simulink model "community_charts"  (R2018a)
settings: Solver=VariableStepAuto  StartTime=0.0  StopTime=1  RelTol=1e-3
settings Model: Creator=86188  LastModifiedBy=86188

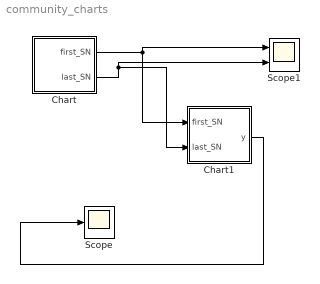
== system community_charts ==
  Chart : Stateflow chart  TreatAsAtomicUnit=on
  Chart1 : Stateflow chart  TreatAsAtomicUnit=on
  Scope : Scope
  Scope1 : Scope  NumInputPorts=2
  wires:
  Chart1/1(y) -> Scope/1
  Chart/2(last_SN) -> Chart1/2(last_SN), Scope1/2
  Chart/1(first_SN) -> Scope1/1, Chart1/1(first_SN)

== matlab function community_charts/Chart1 ==
  settings: executeAtInitialization=1
  data: s function_input; y output =0; first_SN input; last_SN input
function f(s)
  fprintf(s+"\n");

== stateflow chart community_charts/Chart ==
  state add
    en:
    f("en_add")
  (default) -> add : {i=1;first_SN=1;last_SN=0}
  add -> add : [i<=5]
      | {first_SN=1;
      | last_SN=i;i = i + 1}
  data: s function_input; i local; first_SN output; last_SN output
  function f(s):
    | function f(s)
    |   fprintf(s+"\n");
